simulink model "Exp7"  (R2025b)
settings: Solver=VariableStepAuto  StartTime=0.0  StopTime=1000  RelTol=1e-3
libraries: dspfdesign x2
settings Model: Creator=pc  LastModifiedBy=pc

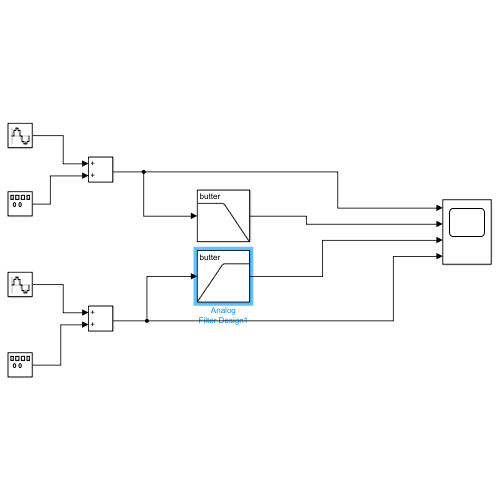
[thumbnail: Simulink's stored preview of the top-level diagram]
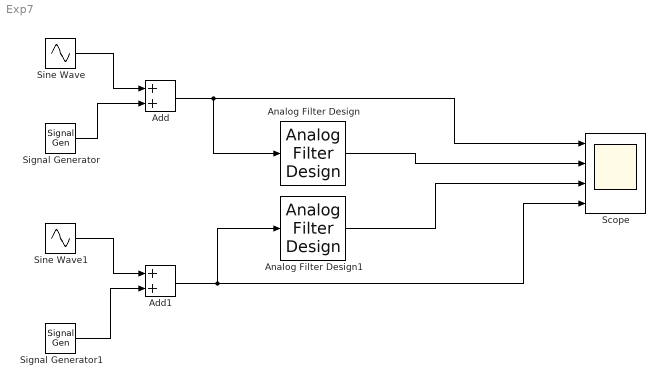
== system Exp7 ==
  Add : Sum
  Add1 : Sum
  Analog Filter Design : dspfdesign/Analog Filter Design  method=Butterworth  filttype=Lowpass  N=8  Wlo=30  Whi=80  Rp=2  Rs=40
  Analog Filter Design1 : dspfdesign/Analog Filter Design  method=Butterworth  filttype=Highpass  N=8  Wlo=10  Whi=80  Rp=2  Rs=40
  Scope : Scope  NumInputPorts=4
      settings: ActiveDisplayYMinimum=-6.2179598478864371  ActiveDisplayYMaximum=6.2408301561321959
  Signal Generator : SignalGenerator  WaveForm=random  Amplitude=2  Frequency=200  Units=rad/sec
  Signal Generator1 : SignalGenerator  WaveForm=random  Amplitude=2  Frequency=100  Units=rad/sec
  Sine Wave : Sin  Amplitude=3  Frequency=50  SampleTime=1
  Sine Wave1 : Sin  Amplitude=3  Frequency=100  SampleTime=1
  wires:
  Sine Wave/1 -> Add/1
  Signal Generator/1 -> Add/2
  Sine Wave1/1 -> Add1/1
  Signal Generator1/1 -> Add1/2
  Add/1 -> Analog Filter Design/1, Scope/1
  Analog Filter Design/1 -> Scope/2
  Analog Filter Design1/1 -> Scope/3
  Add1/1 -> Analog Filter Design1/1, Scope/4
